simulink model "sm_parts_rack_and_pinion"  (R2026a)
settings: Solver=VariableStepAuto  EnableMultiTasking=on
undefined symbols (not defined in the file): Local, X, Y, Z
libraries: Multibody_Parts_Lib x7, sm_lib x6, nesl_utility x1
Description:
  | Copyright 2017-2026 The MathWorks, Inc.
settings Model: Creator=smiller  LastModifiedBy=smiller
settings DebuggingCC: PregeneratedLibrarySubsystemCodeDiagnostic=none
settings SimscapeCC: SimscapeNormalizeSystem=off  SimscapeNominalValues="[{\"value\":\"1\",\"unit\":\"A\"},{\"value\":\"1\",\"unit\":\"bar\"},{\"value\":\"1\",\"unit\":\"cm^2\"},{\"value\":\"1\",\"unit\":\"cm^3/s\"},{\"value\":\"1\",\"unit\":\"kJ/kg\"},{\"value\":\"1\",\"unit\":\"kW\"},{\"value\":\"1\",\"unit\":\"l\"},{\"value\":\"1\",\"unit\":\"N\"},{\"value\":\"1\",\"unit\":\"N*m\"},{\"value\":\"1\",\"unit\":\"V\"}]"
settings ConfigurationSet: Description=SimMechanics 2G
settings ExplorerConfigSet: InternalSimMechanicsExplorerSettings="<ExplorerConfiguration><canonicalview>default</canonicalview><AnimationSetting><BasePlaybackSpeed>1.0</BasePlaybackSpeed><PlaybackSpeedFactor>1.0</PlaybackSpeedFactor></AnimationSetting><TilePanel><TileInfo><Tiles Columns=\"1\" Count=\"1\" Rows=\"1\"><Column Left=\"2\" Weight=\"1\"/><Column Left=\"729\"/><Row Top=\"2\" Weight=\"1\"/><Row Top=\"700\"/><Tile Height=\"1\" Width=\"1\" X=\"0\" Y=\"0\"/></Tiles></TileInfo><SceneInfo><SceneViewer><BGColor><R>1</R><G>1</G><B>1</B></BGColor><Camera><DoPerspective>off</DoPerspective><Position><X>0.69347970485678423</X><Y>0.70143684520355387</Y><Z>0.19040263511746225</Z></Position><Center><X>-0.0046228278298354741</X><Y>-0.0060269620912895006</Y><Z>0.080185507481091212</Z></Center><Up><X>-0.06522973093046347</X><Y>-0.090453491425826038</Y><Z>0.99376216877662316</Z></Up><ViewLimDist>1</ViewLimDist><YLim>0.098536439165472986</YLim><XLim>0.10268383645981076</XLim></Camera></SceneViewer></SceneInfo></TilePanel><MechEditorPanel><Cameras/><GfxPanelCameraMap/><VideoCreator><PlaybackSpeedRatio>1.0</PlaybackSpeedRatio><FrameRate>30</FrameRate><VideoFormat>Motion JPEG AVI</VideoFormat><FrameSize>auto</FrameSize></VideoCreator></MechEditorPanel></ExplorerConfiguration>"

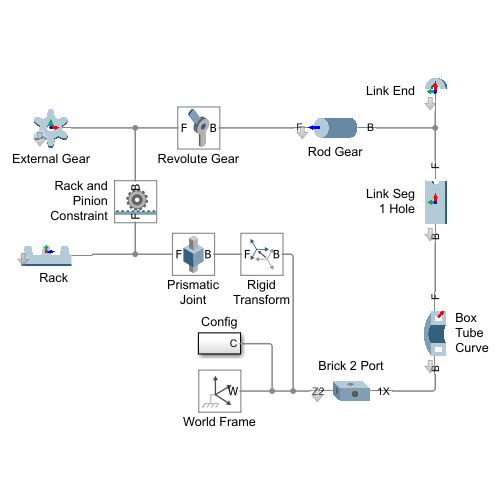
[thumbnail: Simulink's stored preview of the top-level diagram]
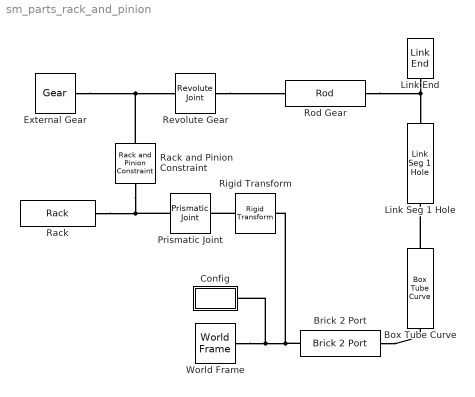
== system sm_parts_rack_and_pinion ==
  Box Tube Curve : Multibody_Parts_Lib/Extrusions/Box Tube Curve  box_ox=0.01  box_ix=0  box_oy=0.025  box_iy=0  arc_rad=0.0125  arc_angle=-90  popup_arcdir=Y  box_rho=7000  box_color=[0 0.4 0.6]  box_opc=1
      settings: SourceProductName=Simscape Multibody Parts Library
  Brick 2 Port : Multibody_Parts_Lib/Basic/Brick 2 Port  len_xyz=[0.0125*2 0.025 0.01]  brick_rho=7000  brick_clr=[0 0.4 0.6]  brick_opc=1  popup_port1=+X  popup_port2=+Z  port1_offset=[0 0 0]
      settings: SourceProductName=Simscape Multibody Parts Library
  Config : Subsystem
  External Gear : Multibody_Parts_Lib/Gears/Gear  popup_gear_type=External  gear_pd=0.125  gear_nt=12  gear_th=0.02  gear_rh=0.005  gear_rt=0.02  gear_rho=7000  gear_clr=[0.8 0.8 0.8]  gear_opc=1  popup_ad_dd=Default  gear_ad=0.125/12  gear_dd=1.157*0.125/12  popup_markings=Two  mark_radius_range=[0.6 0.7]  mark_angle_range=60  mark_color=[1 1 1]*0.2
      settings: SourceProductName=Simscape Multibody Parts Library
  Link End : Multibody_Parts_Lib/Linkages/Link End  circ_radout=0.025/2  circ_radin=0.005  popup_holelr=+X  deg_1=-90  deg_2=90  circ_len=0.01  circ_rho=7000  circ_color=[0 0.4 0.6]  circ_opc=1
      settings: SourceProductName=Simscape Multibody Parts Library
  Link Seg 1 Hole : Multibody_Parts_Lib/Linkages/Link Seg 1 Hole  link_len=0.125/2+0.02+1.157*0.125/12+0.005-0.0125  link_width=0.025  link_radh=0.005  link_holelr=+X  link_thickness=0.01  link_rho=7000  link_color=[0 0.4 0.6]  link_opc=1
      settings: SourceProductName=Simscape Multibody Parts Library
  Prismatic Joint : sm_lib/Joints/Prismatic Joint  JointMode=Normal  CompositeWrenchDir=FollowerOnBase  CompositeWrenchFrame=BaseFrame  SenseConstraintForce=off  SenseConstraintTorque=off  SenseTotalForce=off  SenseTotalTorque=off  PositionTargetSpecify=on  PositionTargetPriority=Low  PositionTargetValue=0  PositionTargetValueUnits=m  VelocityTargetSpecify=off  VelocityTargetPriority=High  VelocityTargetValue=0  VelocityTargetValueUnits=m/s  EquilibriumPosition=0  EquilibriumPositionUnits=m  SpringStiffness=0  SpringStiffnessUnits=N/m  DampingCoefficient=0  DampingCoefficientUnits=N/(m/s)  LowerLimitSpecify=off  LowerLimitBound=-1  LowerLimitBoundUnits=m  LowerLimitStiffness=1e6  LowerLimitStiffnessUnits=N/m  LowerLimitDamping=1e3  LowerLimitDampingUnits=N/(m/s)  LowerLimitTransitionRegionWidth=1e-4  LowerLimitTransitionRegionWidthUnits=m  UpperLimitSpecify=off  UpperLimitBound=1  UpperLimitBoundUnits=m  UpperLimitStiffness=1e6  UpperLimitStiffnessUnits=N/m  UpperLimitDamping=1e3  UpperLimitDampingUnits=N/(m/s)  UpperLimitTransitionRegionWidth=1e-4  UpperLimitTransitionRegionWidthUnits=m  TorqueActuationMode=NoTorque  MotionActuationMode=ComputedMotion  SensePosition=off  SenseVelocity=off  SenseAcceleration=off  SenseTorqueForce=off  SenseLowerLimitTorqueForce=off  SenseUpperLimitTorqueForce=off
  Rack : Multibody_Parts_Lib/Gears/Rack  rack_tp=pi*0.125/12  rack_nt=8  rack_tb=0.02  rack_th=0.02  rack_rho=7000  rack_clr=[0.5 0.5 0.5]  rack_opc=1  popup_ad_dd=Default  rack_ad=0.052/pi  rack_dd=1.157*0.052/pi
      settings: SourceProductName=Simscape Multibody Parts Library
  Rack and Pinion Constraint : sm_lib/Gears and Couplings/Gears/Rack and Pinion Constraint  PinionRadius=0.125/2  PinionRadiusUnits=m  SensingForceTorqueDirection=FollowerOnBase  SensingForceTorqueResolutionFrame=BaseFrame  SenseForce=off  SenseTorque=off
  Revolute Gear : sm_lib/Joints/Revolute Joint  JointMode=Normal  CompositeWrenchDir=FollowerOnBase  CompositeWrenchFrame=BaseFrame  SenseConstraintForce=off  SenseConstraintTorque=off  SenseTotalForce=off  SenseTotalTorque=off  PositionTargetSpecify=off  PositionTargetPriority=High  PositionTargetValue=360/12/2  PositionTargetValueUnits=deg  VelocityTargetSpecify=off  VelocityTargetPriority=High  VelocityTargetValue=0  VelocityTargetValueUnits=deg/s  EquilibriumPosition=0  EquilibriumPositionUnits=deg  SpringStiffness=0  SpringStiffnessUnits=N*m/deg  DampingCoefficient=0  DampingCoefficientUnits=N*m/(deg/s)  LowerLimitSpecify=off  LowerLimitBound=-90  LowerLimitBoundUnits=deg  LowerLimitStiffness=1e4  LowerLimitStiffnessUnits=N*m/deg  LowerLimitDamping=10  LowerLimitDampingUnits=N*m/(deg/s)  LowerLimitTransitionRegionWidth=0.1  LowerLimitTransitionRegionWidthUnits=deg  UpperLimitSpecify=off  UpperLimitBound=90  UpperLimitBoundUnits=deg  UpperLimitStiffness=1e4  UpperLimitStiffnessUnits=N*m/deg  UpperLimitDamping=10  UpperLimitDampingUnits=N*m/(deg/s)  UpperLimitTransitionRegionWidth=0.1  UpperLimitTransitionRegionWidthUnits=deg  TorqueActuationMode=NoTorque  MotionActuationMode=ComputedMotion  SensePosition=off  SenseVelocity=off  SenseAcceleration=off  SenseTorqueForce=off  SenseLowerLimitTorqueForce=off  SenseUpperLimitTorqueForce=off
  Rigid Transform : sm_lib/Frames and Transforms/Rigid Transform  RotationMethod=StandardAxis  FollAlignAxisA=+Z  BaseAlignAxisA=+Y  FollAlignAxisB=+Y  BaseAlignAxisB=+Z  RotationStandardAxis=+X  RotationAngle=90  RotationAngleUnits=deg  RotationArbitraryAxis=[0 0 1]  RotationSequenceAxes=FollowerAxes  RotationSequence=XYX  RotationSequenceAngles=[0 0 0]  RotationSequenceAnglesUnits=deg  RotationMatrix=[1 0 0; 0 1 0; 0 0 1]  Quaternion=[1 0 0 0]  TranslationMethod=StandardAxis  TranslationCartesianOffset=[0 0 0]  TranslationCartesianOffsetUnits=m  TranslationStandardAxis=+Z  TranslationStandardOffset=0.02+1.157*0.125/12  TranslationStandardOffsetUnits=m  TranslationROffset=0  TranslationROffsetUnits=m  TranslationThetaOffset=0  TranslationThetaOffsetUnits=deg  TranslationZOffset=0  TranslationZOffsetUnits=m
  Rod Gear : Multibody_Parts_Lib/Basic/Rod  rod_rad=0.005  rod_len=0.025  rod_rho=7000  rod_color=[0.5 0.5 0.5]  rod_opc=1  popup_zori=Local +Z  popup_markings=None  mark_radius_range=[0.5 1.01]  mark_length_range=1.005  mark_angle_range=30  mark_color=[1 1 1]
      settings: SourceProductName=Simscape Multibody Parts Library
  World Frame : sm_lib/Frames and Transforms/World Frame
  connections:
  External Gear/RConn1 -- Rack and Pinion Constraint/LConn1 -- Revolute Gear/RConn1
  Box Tube Curve/RConn1 -- Link Seg 1 Hole/LConn1
  World Frame/RConn1 -- Config/LConn1 -- Rigid Transform/LConn1 -- Brick 2 Port/RConn1
  Rack and Pinion Constraint/RConn1 -- Rack/RConn1 -- Prismatic Joint/RConn1
  Rigid Transform/RConn1 -- Prismatic Joint/LConn1
  Link End/LConn1 -- Rod Gear/LConn1 -- Link Seg 1 Hole/RConn1
  Revolute Gear/LConn1 -- Rod Gear/RConn1
  Brick 2 Port/LConn1 -- Box Tube Curve/LConn1

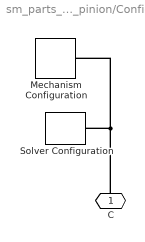
== system sm_parts_rack_and_pinion/Config ==
  Mechanism Configuration : sm_lib/Utilities/Mechanism Configuration  UniformGravity=Constant  GravityVector=[0 -9.80665 0]  GravityVectorUnits=m/s^2  LinearizationDelta=0.001  JointModeTransitionNonlinearIterations=2
  Solver Configuration : nesl_utility/Solver Configuration  PhysicalDomain=network_engine_domain  SubClassName=solver  LeftPortType=input  RightPortType=generic  Tones=[]  Harmonics=[]  SimulateNoise=off  Profile=off  UseLocalSampling=off  EnableSwitchedLinearOptims=on  FrequencyDomain=off  UseCCode=off  RelTol=0.001  AbsTol=1e-06  MinStep=1e-09  ToWorkspace=off  RevertToSquareIcSolve=off  NumHomotopyIterations=100  PhasorMode=off  PhasorModeNumHarmonics=1  ConsistencySolver=NEWTON_FTOL  CanonicalOrdering=UNORDERED  OptimizeIntermediates=UNOPTIMIZED  IndexReductionMethod=DerivativeReplacement  DoDC=off  ResidualTolerance=1e-09  ConsistencyTolSource=GLOBAL  ConsistencyAbsTol=0.001  ConsistencyRelTol=0.001  ConsistencyTolFactor=0.001  UseLocalSolver=off  LocalSolverChoice=NE_BACKWARD_EULER_ADVANCER  ResolveIndetEquations=on  FunctionEvalNumThread=1  LocalSolverSampleTime=0.001  DoFixedCost=off  MaxNonlinIter=3  MaxModeIter=2  ComputeImpulses=off  ImpulseIterations=2  LinearAlgebra=Sparse  LinearAlgebraNumThread=0  EquationFormulation=NE_TIME_EF  DelaysMemoryBudget=1024  AutomaticFiltering=on  FilteringTimeConstant=0.001  PartitionStorageMethod=AS_NEEDED  PartitionMemoryBudget=1024  PartitionMethod=FAST  MultibodyUseLocalSolver=off  MultibodyLocalSolverChoice=ODE1  MultibodyLocalSolverSampleTime=0.001
  C : PMIOPort  Side=Left
  connections:
  Mechanism Configuration/RConn1 -- C/RConn1 -- Solver Configuration/RConn1
